simulink model "chap8_4sim"  (R2015a)
settings: Solver=ode45  StartTime=0.0  StopTime=30  RelTol=1e-3
settings Model: Creator=zhr  LastModifiedBy=zhr

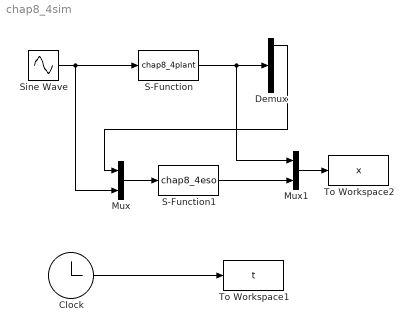
== system chap8_4sim ==
  Clock : Clock
  Demux : Demux  Outputs=3
  Mux : Mux  Inputs=2
  Mux1 : Mux  Inputs=2
  S-Function : S-Function  FunctionName=chap8_4plant
  S-Function1 : S-Function  FunctionName=chap8_4eso
  Sine Wave : Sin  Frequency=2*pi/7  SampleTime=0
  To Workspace1 : ToWorkspace  VariableName=t  SampleTime=-1
  To Workspace2 : ToWorkspace  VariableName=x  SampleTime=-1
  wires:
  Clock/1 -> To Workspace1/1
  Sine Wave/1 -> Mux/2, S-Function/1
  S-Function/1 -> Mux1/1, Demux/1
  Demux/1 -> Mux/1
  Mux/1 -> S-Function1/1
  S-Function1/1 -> Mux1/2
  Mux1/1 -> To Workspace2/1
